simulink model "Model_Compare"  (R2018a)
settings: Solver=FixedStepDiscrete  StartTime=0.0  StopTime=37  FixedStep=Ts  RelTol=1e-3  EnableMultiTasking=on
values from neighbouring files (symbols this model uses):
  alpha_f0 = states(7)    [IS_2impulse.m]    (also in IS_3impulse.m; IS_4impulse.m; InputShaper.m; InputShaper2.m = 0)
  alpha_r0 = states(8)    [IS_2impulse.m]    (also in IS_3impulse.m; IS_4impulse.m; InputShaper.m; InputShaper2.m = 0)
  Bx_ash_f = 11.7    [ISData.m]    (also in SbWdata.m; pacjeka_params.m)
  Bx_ash_r = 11.1    [ISData.m]    (also in SbWdata.m; pacjeka_params.m)
  Bx_snow_f = 10.2    [ISData.m]    (also in SbWdata.m; pacjeka_params.m)
  Bx_snow_r = 9.71    [ISData.m]    (also in SbWdata.m; pacjeka_params.m)
  Bx_wash_f = 12    [ISData.m]    (also in SbWdata.m; pacjeka_params.m)
  Bx_wash_r = 11.5    [ISData.m]    (also in SbWdata.m; pacjeka_params.m)
  By_ash_f = 8.86    [ISData.m]    (also in SbWdata.m; pacjeka_params.m)
  By_ash_r = 9.30    (= 9.3)    [ISData.m]    (also in SbWdata.m; pacjeka_params.m)
  By_snow_f = 19.1    [ISData.m]    (also in SbWdata.m; pacjeka_params.m)
  By_snow_r = 20.0    (= 20)    [ISData.m]    (also in SbWdata.m; pacjeka_params.m)
  By_wash_f = 10.7    [ISData.m]    (also in SbWdata.m; pacjeka_params.m)
  By_wash_r = 11.3    [ISData.m]    (also in SbWdata.m; pacjeka_params.m)
  Cx_ash_f = 1.69    [ISData.m]    (also in SbWdata.m; pacjeka_params.m)
  Cx_ash_r = 1.69    [ISData.m]    (also in SbWdata.m; pacjeka_params.m)
  Cx_snow_f = 1.96    [ISData.m]    (also in SbWdata.m; pacjeka_params.m)
  Cx_snow_r = 1.96    [ISData.m]    (also in SbWdata.m; pacjeka_params.m)
  Cx_wash_f = 1.80    (= 1.8)    [ISData.m]    (also in SbWdata.m; pacjeka_params.m)
  Cx_wash_r = 1.80    (= 1.8)    [ISData.m]    (also in SbWdata.m; pacjeka_params.m)
  Cy_ash_f = 1.19    [ISData.m]    (also in SbWdata.m; pacjeka_params.m)
  Cy_ash_r = 1.19    [ISData.m]    (also in SbWdata.m; pacjeka_params.m)
  Cy_snow_f = 0.550    (= 0.55)    [ISData.m]    (also in SbWdata.m; pacjeka_params.m)
  Cy_snow_r = 0.550    (= 0.55)    [ISData.m]    (also in SbWdata.m; pacjeka_params.m)
  Cy_wash_f = 1.07    [ISData.m]    (also in SbWdata.m; pacjeka_params.m)
  Cy_wash_r = 1.07    [ISData.m]    (also in SbWdata.m; pacjeka_params.m)
  D_phi = 16000    [ISData.m]    (also in IS_2impulse.m; IS_3impulse.m; IS_4impulse.m; InputShaper.m)
  D_theta = 30960    [ISData.m]    (also in IS_2impulse.m; IS_3impulse.m; IS_4impulse.m; InputShaper.m)
  delta_r = 0    [ISData.m]    (also in IS_2impulse.m; IS_3impulse.m; IS_4impulse.m; InputShaper.m)
  epsilon = 0.4    [ISData.m]    (also in IS_2impulse.m; IS_3impulse.m; IS_4impulse.m; InputShaper.m)
  Ex_ash_f = 0.377    [ISData.m]    (also in SbWdata.m; pacjeka_params.m)
  Ex_ash_r = 0.362    [ISData.m]    (also in SbWdata.m; pacjeka_params.m)
  Ex_snow_f = 0.651    [ISData.m]    (also in SbWdata.m; pacjeka_params.m)
  Ex_snow_r = 0.624    [ISData.m]    (also in SbWdata.m; pacjeka_params.m)
  Ex_wash_f = 0.313    [ISData.m]    (also in SbWdata.m; pacjeka_params.m)
  Ex_wash_r = 0.300    (= 0.3)    [ISData.m]    (also in SbWdata.m; pacjeka_params.m)
  Ey_ash_f = -1.21    [ISData.m]    (also in SbWdata.m; pacjeka_params.m)
  Ey_ash_r = -1.11    [ISData.m]    (also in SbWdata.m; pacjeka_params.m)
  Ey_snow_f = -2.1    [ISData.m]    (also in SbWdata.m; pacjeka_params.m)
  Ey_snow_r = -1.93    [ISData.m]    (also in SbWdata.m; pacjeka_params.m)
  Ey_wash_f = -2.14    [ISData.m]    (also in SbWdata.m; pacjeka_params.m)
  Ey_wash_r = -1.97    [ISData.m]    (also in SbWdata.m; pacjeka_params.m)
  g = 9.81    [ISData.m]    (also in IS_2impulse.m; IS_3impulse.m; IS_4impulse.m; InputShaper.m)
  h = 0.5    [ISData.m]    (also in IS_2impulse.m; IS_3impulse.m; IS_4impulse.m; InputShaper.m)
  Iw = 4    [ISData.m]    (also in IS_2impulse.m; IS_3impulse.m; IS_4impulse.m; InputShaper.m)
  Ixx = 602.1923    [ISData.m]    (also in IS_2impulse.m; IS_3impulse.m; IS_4impulse.m; InputShaper.m)
  Iyy = 2.7370e+03    (= 2737)    [ISData.m]    (also in IS_2impulse.m; IS_3impulse.m; IS_4impulse.m; InputShaper.m)
  Iz = Izz    (= 3070)    [IS_2impulse.m]    (also in IS_3impulse.m; IS_4impulse.m; InputShaper.m; InputShaper2.m)
  Izz = 3070    [ISData.m]    (also in IS_2impulse.m; IS_3impulse.m; IS_4impulse.m; InputShaper.m)
  K_phi = 178000    [ISData.m]    (also in IS_2impulse.m; IS_3impulse.m; IS_4impulse.m; InputShaper.m)
  K_theta = 363540    [ISData.m]    (also in IS_2impulse.m; IS_3impulse.m; IS_4impulse.m; InputShaper.m)
  l = l_f+l_r    (= 2.67)    [IS_2impulse.m]    (also in IS_3impulse.m; IS_4impulse.m; InputShaper.m; InputShaper2.m)
  l_f = 1.2110    (= 1.211)    [ISData.m]    (also in IS_2impulse.m; IS_3impulse.m; IS_4impulse.m; InputShaper.m)
  l_r = 1.4590    (= 1.459)    [ISData.m]    (also in IS_2impulse.m; IS_3impulse.m; IS_4impulse.m; InputShaper.m)
  m = 1830    [ISData.m]    (also in IS_2impulse.m; IS_3impulse.m; IS_4impulse.m; InputShaper.m)
  mu_x_ash_f = 1.20    (= 1.2)    [ISData.m]    (also in SbWdata.m; pacjeka_params.m)
  mu_x_ash_r = 1.20    (= 1.2)    [ISData.m]    (also in SbWdata.m; pacjeka_params.m)
  mu_x_snow_f = 0.407    [ISData.m]    (also in SbWdata.m; pacjeka_params.m)
  mu_x_snow_r = 0.409    [ISData.m]    (also in SbWdata.m; pacjeka_params.m)
  mu_x_wash_f = 1.06    [ISData.m]    (also in SbWdata.m; pacjeka_params.m)
  mu_x_wash_r = 1.07    [ISData.m]    (also in SbWdata.m; pacjeka_params.m)
  mu_y_ash_f = 0.935    [ISData.m]    (also in SbWdata.m; pacjeka_params.m)
  mu_y_ash_r = 0.961    [ISData.m]    (also in SbWdata.m; pacjeka_params.m)
  mu_y_snow_f = 0.383    [ISData.m]    (also in SbWdata.m; pacjeka_params.m)
  mu_y_snow_r = 0.394    [ISData.m]    (also in SbWdata.m; pacjeka_params.m)
  mu_y_wash_f = 0.885    [ISData.m]    (also in SbWdata.m; pacjeka_params.m)
  mu_y_wash_r = 0.911    [ISData.m]    (also in SbWdata.m; pacjeka_params.m)
  omega0 = Vx0/Rw    (= 48.6005830904)    [ISData.m]    (also in IS_2impulse.m = 74.1; IS_3impulse.m = 74.1; IS_4impulse.m = 74.1; InputShaper.m = 55.5666666667)
  omega_f0 = states(5)    [IS_2impulse.m]    (also in IS_3impulse.m; IS_4impulse.m; InputShaper.m; InputShaper2.m = 55.5666666667)
  omega_r0 = states(6)    [IS_2impulse.m]    (also in IS_3impulse.m; IS_4impulse.m; InputShaper.m; InputShaper2.m = 55.5666666667)
  psi0 = states(2)    [IS_2impulse.m]    (also in IS_3impulse.m; IS_4impulse.m; InputShaper.m; InputShaper2.m = 0)
  psi_dot0 = states(1)    [IS_2impulse.m]    (also in IS_3impulse.m; IS_4impulse.m; InputShaper.m; InputShaper2.m = 0)
  Px0 = states(9)    [IS_2impulse.m]    (also in IS_3impulse.m; IS_4impulse.m; InputShaper.m; InputShaper2.m = 0)
  Py0 = states(10)    [IS_2impulse.m]    (also in IS_3impulse.m; IS_4impulse.m; InputShaper.m; InputShaper2.m = 0)
  Re = Rw    (= 0.3)    [IS_2impulse.m]    (also in IS_3impulse.m; IS_4impulse.m; InputShaper.m; InputShaper2.m)
  road = 1    [ISData.m]    (also in IS_2impulse.m; IS_3impulse.m; IS_4impulse.m; InputShaper.m)
  Rw = 0.3430    (= 0.343)    [ISData.m]    (also in IS_2impulse.m = 0.3; IS_3impulse.m = 0.3; IS_4impulse.m = 0.3; InputShaper.m = 0.3)
  sigma = epsilon    (= 0.4)    [IS_2impulse.m]    (also in IS_3impulse.m; IS_4impulse.m; InputShaper.m; InputShaper2.m)
  Ts = 0.001    [ISData.m]    (also in IS_2impulse.m; IS_3impulse.m; IS_4impulse.m; InputShaper.m)
  Tsmall = 0.001    [ISData.m]    (also in IS_2impulse.m; IS_3impulse.m; IS_4impulse.m; InputShaper.m)
  Vx0 = 16.67    [ISData.m]    (also in IS_2impulse.m = states(3); IS_3impulse.m = states(3); IS_4impulse.m = states(3); InputShaper.m = states(3))
  Vy0 = states(4)    [IS_2impulse.m]    (also in IS_3impulse.m; IS_4impulse.m; InputShaper.m; InputShaper2.m = 0)
  w = 0.7700    (= 0.77)    [ISData.m]    (also in IS_2impulse.m; IS_3impulse.m; IS_4impulse.m; InputShaper.m)
undefined symbols (not defined in the file or in its folder): theta_sw_FH
libraries: simulink x2
(part 3 of 3)

== system Model_Compare/3DoF_Vehicle1/Subsystem1/Pacjeka_parameters_Subsystem/WetAshphalt_condition_subsystem ==
  Action Port : ActionPort  ActionType=case
  Bx_wash_f : Constant  Value=Bx_wash_f
  Bx_wash_r : Constant  Value=Bx_wash_r
  By_wash_f : Constant  Value=By_wash_f
  By_wash_r : Constant  Value=By_wash_r
  Cx_wash_f : Constant  Value=Cx_wash_f
  Cx_wash_r : Constant  Value=Cx_wash_r
  Cy_wash_f : Constant  Value=Cy_wash_f
  Cy_wash_r : Constant  Value=Cy_wash_r
  Ex_wash_f : Constant  Value=Ex_wash_f
  Ex_wash_r : Constant  Value=Ex_wash_r
  Ey_wash_f : Constant  Value=Ey_wash_f
  Ey_wash_r : Constant  Value=Ey_wash_r
  Mux : Mux  Inputs=16
      settings: DisplayOption=signals
  mu_x_wash_f : Constant  Value=mu_x_wash_f
  mu_x_wash_r : Constant  Value=mu_x_wash_r
  mu_y_wash_f : Constant  Value=mu_y_wash_f
  mu_y_wash_r : Constant  Value=mu_y_wash_r
  Out1 : Outport  OutDataTypeStr=double  SampleTime=Ts
  wires:
  mu_x_wash_f/1 -> Mux/1  "mu_x_wash_f"
  mu_y_wash_f/1 -> Mux/2  "mu_y_wash_f"
  Cx_wash_f/1 -> Mux/3  "Cx_wash_f"
  Cy_wash_f/1 -> Mux/4  "Cy_wash_f"
  Bx_wash_f/1 -> Mux/5  "Bx_wash_f"
  By_wash_f/1 -> Mux/6  "By_wash_f"
  Ex_wash_f/1 -> Mux/7  "Ex_wash_f"
  Ey_wash_f/1 -> Mux/8  "E_y_wash_f"
  Cy_wash_r/1 -> Mux/12  "Cy_wash_r"
  Cx_wash_r/1 -> Mux/11  "Cx_wash_r"
  By_wash_r/1 -> Mux/14  "By_wash_r"
  Bx_wash_r/1 -> Mux/13  "Bx_wash_r"
  mu_y_wash_r/1 -> Mux/10  "mu_y_wash_r"
  Ex_wash_r/1 -> Mux/15  "Ex_wash_r"
  mu_x_wash_r/1 -> Mux/9  "mu_x_wash_r"
  Ey_wash_r/1 -> Mux/16  "Ey_wash_r"
  Mux/1 -> Out1/1

== system Model_Compare/3DoF_Vehicle1/Subsystem1/Vxdot_subsystem/Fy_subsystem ==
  Fyf : Inport
  Fxf : Inport  Port=2
  Fxr : Inport  Port=3
  cosDelta : Inport  Port=4
  sinDelta : Inport  Port=5
  Add : Sum
  Mux : Mux  Inputs=3
  Terminator : Terminator
  Fx : Outport
  wires:
  Add/1 -> Fx/1
  Fxf/1 -> Add/1
  Fxr/1 -> Add/2
  Mux/1 -> Terminator/1
  cosDelta/1 -> Mux/1
  sinDelta/1 -> Mux/2
  Fyf/1 -> Mux/3

== system Model_Compare/3DoF_Vehicle1/Subsystem1/Vydot_subsystem/Fy_subsystem ==
  Fyf : Inport
  Fyr : Inport  Port=2
  Fxf : Inport  Port=3
  cosDelta : Inport  Port=4
  sinDelta : Inport  Port=5
  Add : Sum  Inputs=2
  Mux : Mux  Inputs=3
  Terminator : Terminator
  Fy : Outport
  wires:
  Add/1 -> Fy/1
  Fyf/1 -> Add/1
  Fyr/1 -> Add/2
  Fxf/1 -> Mux/1
  cosDelta/1 -> Mux/2
  sinDelta/1 -> Mux/3
  Mux/1 -> Terminator/1

== system Model_Compare/Vehicle_Sim/Vehicle_model/Fz_Subsystem/tau_phi_subsystem ==
  K_phi : Inport
  D_phi : Inport  Port=2
  phi_dot : Inport  Port=3
  phi : Inport  Port=4
  Add : Sum
  Add1 : Sum
  Divide{,1..3} (4 alike) : Product  Inputs=**
  Gain : Gain  Gain=0.5
  Gain1 : Gain  Gain=0.5
  tau_phi_f : Outport
  tau_phi_r : Outport  Port=2
  wires:
  Divide2/1 -> Add1/1
  Divide/1 -> Add/1
  Add/1 -> tau_phi_f/1  "tau_phi_f"
  Divide1/1 -> Add/2
  Gain1/1 -> Divide3/1, Divide1/1  "D_phi_r"
  Gain/1 -> Divide2/1, Divide/1  "K_phi_r"
  D_phi/1 -> Gain1/1
  phi/1 -> Divide2/2, Divide/2  "phi"
  Divide3/1 -> Add1/2
  phi_dot/1 -> Divide3/2, Divide1/2  "phi_dot"
  K_phi/1 -> Gain/1
  Add1/1 -> tau_phi_r/1  "tau_phi_r"

== system Model_Compare/Vehicle_Sim/Vehicle_model/Fz_Subsystem/tau_theta_subsystem ==
  theta_dot : Inport  OutDataTypeStr=double  SampleTime=Ts  LockScale=on
  theta : Inport  Port=2  OutDataTypeStr=double  SampleTime=Ts
  K_theta : Inport  Port=3  OutDataTypeStr=double  SampleTime=Ts
  D_theta : Inport  Port=4  OutDataTypeStr=double  SampleTime=Ts
  Add : Sum
  Divide : Product  Inputs=**
  Divide1 : Product  Inputs=**
  tau_theta : Outport  OutDataTypeStr=double  SampleTime=Ts
  wires:
  Add/1 -> tau_theta/1
  Divide/1 -> Add/1
  Divide1/1 -> Add/2
  K_theta/1 -> Divide/1
  D_theta/1 -> Divide1/2
  theta_dot/1 -> Divide1/1
  theta/1 -> Divide/2

== system Model_Compare/Vehicle_Sim/Vehicle_model/Pacjeka_parameters_Subsystem/Ashphalt_condition_subsystem ==
  Action Port : ActionPort  ActionType=then
  Bx_ash_f : Constant  Value=Bx_ash_f
  Bx_ash_r : Constant  Value=Bx_ash_r
  By_ash_f : Constant  Value=By_ash_f
  By_ash_r : Constant  Value=By_ash_r
  Cx_ash_f : Constant  Value=Cx_ash_f
  Cx_ash_r : Constant  Value=Cx_ash_r
  Cy_ash_f : Constant  Value=Cy_ash_f
  Cy_ash_r : Constant  Value=Cy_ash_r
  Ex_ash_f : Constant  Value=Ex_ash_f
  Ex_ash_r : Constant  Value=Ex_ash_r
  Ey_ash_f : Constant  Value=Ey_ash_f
  Ey_ash_r : Constant  Value=Ey_ash_r
  Mux : Mux  Inputs=16
      settings: DisplayOption=signals
  mu_x_ash_f : Constant  Value=mu_x_ash_f
  mu_x_ash_r : Constant  Value=mu_x_ash_r
  mu_y_ash_f : Constant  Value=mu_y_ash_f
  mu_y_ash_r : Constant  Value=mu_y_ash_r
  Out1 : Outport  OutDataTypeStr=double  SampleTime=Ts
  wires:
  mu_x_ash_f/1 -> Mux/1  "mu_x_ash_f"
  mu_y_ash_f/1 -> Mux/2  "mu_y_ash_f"
  Cx_ash_f/1 -> Mux/3  "Cx_ash_f"
  Cy_ash_f/1 -> Mux/4  "Cy_ash_f"
  Bx_ash_f/1 -> Mux/5  "Bx_ash_f"
  By_ash_f/1 -> Mux/6  "By_ash_f"
  Ex_ash_f/1 -> Mux/7  "Ex_ash_f"
  Ey_ash_f/1 -> Mux/8  "E_y_ash_f"
  Cy_ash_r/1 -> Mux/12  "Cy_ash_r"
  Cx_ash_r/1 -> Mux/11  "Cx_ash_r"
  By_ash_r/1 -> Mux/14  "By_ash_r"
  Bx_ash_r/1 -> Mux/13  "Bx_ash_r"
  mu_y_ash_r/1 -> Mux/10  "mu_y_ash_r"
  Ex_ash_r/1 -> Mux/15  "Ex_ash_r"
  mu_x_ash_r/1 -> Mux/9  "mu_x_ash_r"
  Ey_ash_r/1 -> Mux/16  "Ey_ash_r"
  Mux/1 -> Out1/1

== system Model_Compare/Vehicle_Sim/Vehicle_model/Pacjeka_parameters_Subsystem/Snow_condition_subsystem ==
  Action Port : ActionPort  ActionType=else
  Bx_snow_f : Constant  Value=Bx_snow_f
  Bx_snow_r : Constant  Value=Bx_snow_r
  By_snow_f : Constant  Value=By_snow_f
  By_snow_r : Constant  Value=By_snow_r
  Cx_snow_f : Constant  Value=Cx_snow_f
  Cx_snow_r : Constant  Value=Cx_snow_r
  Cy_snow_f : Constant  Value=Cy_snow_f
  Cy_snow_r : Constant  Value=Cy_snow_r
  Ex_snow_f : Constant  Value=Ex_snow_f
  Ex_snow_r : Constant  Value=Ex_snow_r
  Ey_snow_f : Constant  Value=Ey_snow_f
  Ey_snow_r : Constant  Value=Ey_snow_r
  Mux : Mux  Inputs=16
  mu_x_snow_f : Constant  Value=mu_x_snow_f
  mu_x_snow_r : Constant  Value=mu_x_snow_r
  mu_y_snow_f : Constant  Value=mu_y_snow_f
  mu_y_snow_r : Constant  Value=mu_y_snow_r
  Out1 : Outport  OutDataTypeStr=double  SampleTime=Ts
  wires:
  Ex_snow_r/1 -> Mux/15
  Cy_snow_r/1 -> Mux/12
  By_snow_r/1 -> Mux/14
  Cx_snow_r/1 -> Mux/11
  mu_y_snow_r/1 -> Mux/10
  mu_x_snow_r/1 -> Mux/9
  Bx_snow_r/1 -> Mux/13
  Ey_snow_r/1 -> Mux/16
  mu_x_snow_f/1 -> Mux/1
  mu_y_snow_f/1 -> Mux/2
  Cx_snow_f/1 -> Mux/3
  Cy_snow_f/1 -> Mux/4
  Bx_snow_f/1 -> Mux/5
  By_snow_f/1 -> Mux/6
  Ex_snow_f/1 -> Mux/7
  Ey_snow_f/1 -> Mux/8
  Mux/1 -> Out1/1

== system Model_Compare/Vehicle_Sim/Vehicle_model/omega_alpha_and_k_values_subsystem/Subsystem ==
  Vx1 : Inport  OutDataTypeStr=double  SampleTime=Ts
  Vy1 : Inport  Port=2  OutDataTypeStr=double  SampleTime=Ts
  epsilon : Inport  Port=3  OutDataTypeStr=double  SampleTime=Ts
  apha_f1_curr : Inport  Port=4  OutDataTypeStr=double  SampleTime=Tsmall
  Add : Sum  Inputs=+-
  Add1 : Sum
  Divide : Product  Inputs=*/
  Divide1 : Product  Inputs=*/
  Gain : Gain  Gain=-1
  Gain1 : Gain  Gain=Tsmall
  Product : Product
  Product1 : Product
  Trigonometric Function : Trigonometry  Operator=atan
  alpha_f1_next : Outport  OutDataTypeStr=double  SampleTime=Tsmall
  wires:
  Gain1/1 -> Add1/1  "alpha_f1dot*Tsmall"
  Vx1/1 -> Divide1/2, Divide/1
  Product1/1 -> Add/2
  Divide1/1 -> Trigonometric Function/1
  Divide/1 -> Gain/1, Product1/1
  Product/1 -> Add/1
  epsilon/1 -> Divide/2
  Trigonometric Function/1 -> Product/2
  Vy1/1 -> Divide1/1
  Add/1 -> Gain1/1  "alpha_f1_dot"
  Gain/1 -> Product/1
  Add1/1 -> alpha_f1_next/1
  apha_f1_curr/1 -> Add1/2, Product1/2

== system Model_Compare/Vehicle_Sim/Vehicle_model/omega_alpha_and_k_values_subsystem/Subsystem1 ==
  Vx2 : Inport  OutDataTypeStr=double  SampleTime=Ts
  Vy2 : Inport  Port=2  OutDataTypeStr=double  SampleTime=Ts
  epsilon : Inport  Port=3  OutDataTypeStr=double  SampleTime=Ts
  alpha_f2_curr : Inport  Port=4  OutDataTypeStr=double  SampleTime=Tsmall
  Add : Sum  Inputs=+-
  Add1 : Sum
  Divide : Product  Inputs=*/
  Divide1 : Product  Inputs=*/
  Gain : Gain  Gain=-1
  Gain1 : Gain  Gain=Tsmall
  Product : Product
  Product1 : Product
  Trigonometric Function : Trigonometry  Operator=atan
  alpha_f2_next : Outport  OutDataTypeStr=double  SampleTime=Tsmall
  wires:
  Gain1/1 -> Add1/1  "alpha_f2dot*Tsmall"
  Vx2/1 -> Divide1/2, Divide/1
  Product1/1 -> Add/2
  Divide1/1 -> Trigonometric Function/1
  Divide/1 -> Gain/1, Product1/1
  Product/1 -> Add/1
  epsilon/1 -> Divide/2
  Trigonometric Function/1 -> Product/2
  Vy2/1 -> Divide1/1
  Add/1 -> Gain1/1  "alpha_f2_dot"
  Gain/1 -> Product/1
  alpha_f2_curr/1 -> Add1/2, Product1/2
  Add1/1 -> alpha_f2_next/1

== system Model_Compare/Vehicle_Sim/Vehicle_model/omega_alpha_and_k_values_subsystem/Subsystem2 ==
  Vx3 : Inport  OutDataTypeStr=double  SampleTime=Ts
  Vy3 : Inport  Port=2  OutDataTypeStr=double  SampleTime=Ts
  epsilon : Inport  Port=3  OutDataTypeStr=double  SampleTime=Ts
  alpha_r3_curr : Inport  Port=4  OutDataTypeStr=double  SampleTime=Tsmall
  Add : Sum  Inputs=+-
  Add1 : Sum
  Divide : Product  Inputs=*/
  Divide1 : Product  Inputs=*/
  Gain : Gain  Gain=-1
  Gain1 : Gain  Gain=Tsmall
  Product : Product
  Product1 : Product
  Trigonometric Function : Trigonometry  Operator=atan
  alpha_r3_next : Outport  OutDataTypeStr=double  SampleTime=Tsmall
  wires:
  Gain1/1 -> Add1/1  "alpha_r3dot*Tsmall"
  Vx3/1 -> Divide1/2, Divide/1
  Product1/1 -> Add/2
  Divide1/1 -> Trigonometric Function/1
  Divide/1 -> Gain/1, Product1/1
  Product/1 -> Add/1
  epsilon/1 -> Divide/2
  Trigonometric Function/1 -> Product/2
  Vy3/1 -> Divide1/1
  Add/1 -> Gain1/1  "alpha_r3_dot"
  Gain/1 -> Product/1
  alpha_r3_curr/1 -> Add1/2, Product1/2
  Add1/1 -> alpha_r3_next/1

== system Model_Compare/Vehicle_Sim/Vehicle_model/omega_alpha_and_k_values_subsystem/Subsystem3 ==
  Vx4 : Inport  OutDataTypeStr=double  SampleTime=Ts
  Vy4 : Inport  Port=2  OutDataTypeStr=double  SampleTime=Ts
  epsilon : Inport  Port=3  OutDataTypeStr=double  SampleTime=Ts
  alpha_r4_curr : Inport  Port=4  OutDataTypeStr=double  SampleTime=Tsmall
  Add : Sum  Inputs=+-
  Add1 : Sum
  Divide : Product  Inputs=*/
  Divide1 : Product  Inputs=*/
  Gain : Gain  Gain=-1
  Gain1 : Gain  Gain=Tsmall
  Product : Product
  Product1 : Product
  Trigonometric Function : Trigonometry  Operator=atan
  alpha_r4_next : Outport  OutDataTypeStr=double  SampleTime=Tsmall
  wires:
  Gain1/1 -> Add1/1  "alpha_r4dot*Tsmall"
  Vx4/1 -> Divide1/2, Divide/1
  Product1/1 -> Add/2
  Divide1/1 -> Trigonometric Function/1
  Divide/1 -> Gain/1, Product1/1
  Product/1 -> Add/1
  epsilon/1 -> Divide/2
  Trigonometric Function/1 -> Product/2
  Vy4/1 -> Divide1/1
  Add/1 -> Gain1/1  "alpha_r4_dot"
  Gain/1 -> Product/1
  alpha_r4_curr/1 -> Add1/2, Product1/2
  Add1/1 -> alpha_r4_next/1

== system Model_Compare/Vehicle_Sim/Vehicle_model/omega_alpha_and_k_values_subsystem/Subsystem4 ==
  T1 : Inport  OutDataTypeStr=double  SampleTime=Ts
  T2 : Inport  Port=2  OutDataTypeStr=double  SampleTime=Ts
  T3 : Inport  Port=3  OutDataTypeStr=double  SampleTime=Ts
  T4 : Inport  Port=4  OutDataTypeStr=double  SampleTime=Ts
  Iw : Inport  Port=5  OutDataTypeStr=double  SampleTime=Ts
  Fx1 : Inport  Port=6  OutDataTypeStr=double  SampleTime=Ts
  Fx2 : Inport  Port=7  OutDataTypeStr=double  SampleTime=Ts
  Fx3 : Inport  Port=8  OutDataTypeStr=double  SampleTime=Ts
  Fx4 : Inport  Port=9  OutDataTypeStr=double  SampleTime=Ts
  Rw : Inport  Port=10  OutDataTypeStr=double  SampleTime=Ts
  Add{4..7} (4 alike) : Sum  Inputs=+-
  Divide{4..7} (4 alike) : Product  Inputs=*/
  Product{4..7} (4 alike) : Product
  omega_dot1 : Outport  OutDataTypeStr=double  SampleTime=Tsmall
  omega_dot2 : Outport  Port=2  OutDataTypeStr=double  SampleTime=Tsmall
  omega_dot3 : Outport  Port=3  OutDataTypeStr=double  SampleTime=Tsmall
  omega_dot4 : Outport  Port=4  OutDataTypeStr=double  SampleTime=Tsmall
  wires:
  Product7/1 -> Add7/2
  Add7/1 -> Divide7/1
  Iw/1 -> Divide7/2, Divide6/2, Divide5/2, Divide4/2
  Add5/1 -> Divide5/1
  T1/1 -> Add4/1
  Product5/1 -> Add5/2
  Rw/1 -> Product4/2, Product5/2, Product7/2, Product6/2
  Divide7/1 -> omega_dot4/1  "omega_dot4"
  Fx3/1 -> Product6/1
  Add4/1 -> Divide4/1
  Fx2/1 -> Product5/1
  T4/1 -> Add7/1
  Fx1/1 -> Product4/1
  T3/1 -> Add6/1
  Product4/1 -> Add4/2
  T2/1 -> Add5/1
  Product6/1 -> Add6/2
  Add6/1 -> Divide6/1
  Fx4/1 -> Product7/1
  Divide6/1 -> omega_dot3/1  "omega_dot3"
  Divide5/1 -> omega_dot2/1  "omega_dot2"
  Divide4/1 -> omega_dot1/1  "omega_dot1"

== system Model_Compare/Vehicle_Sim/Vehicle_model/omega_alpha_and_k_values_subsystem/Subsystem5 ==
  Vx : Inport  OutDataTypeStr=double  SampleTime=Ts
  w : Inport  Port=2  OutDataTypeStr=double  SampleTime=Ts
  delta_f2 : Inport  Port=3  OutDataTypeStr=double  SampleTime=Ts
  Vy : Inport  Port=4  OutDataTypeStr=double  SampleTime=Ts
  l_f : Inport  Port=5  OutDataTypeStr=double  SampleTime=Ts
  l_r : Inport  Port=6  OutDataTypeStr=double  SampleTime=Ts
  psi_dot : Inport  Port=7  OutDataTypeStr=double  SampleTime=Ts
  Add : Sum
  Add1 : Sum
  Add2 : Sum  Inputs=-+
  Constant : Constant  Value=delta_r
  Cos : Trigonometry  Operator=cos
  Cos1 : Trigonometry  Operator=cos
  Gain{,1..3} (4 alike) : Gain
  Multiply : Product
  Multiply1 : Product
  Multiply2 : Product
  Subsystem : Subsystem
  Subsystem1 : Subsystem
  Subsystem2 : Subsystem
  Subsystem3 : Subsystem
  Subtract : Sum  Inputs=+-
  sin : Trigonometry
  sin1 : Trigonometry
  Vx1 : Outport  OutDataTypeStr=double  SampleTime=Ts
  Vx2 : Outport  Port=2  OutDataTypeStr=double  SampleTime=Ts
  Vx3 : Outport  Port=3  OutDataTypeStr=double  SampleTime=Ts
  Vx4 : Outport  Port=4  OutDataTypeStr=double  SampleTime=Ts
  Vy1 : Outport  Port=5  OutDataTypeStr=double  SampleTime=Ts
  Vy2 : Outport  Port=6  OutDataTypeStr=double  SampleTime=Ts
  Vy3 : Outport  Port=7  OutDataTypeStr=double  SampleTime=Ts
  Vy4 : Outport  Port=8  OutDataTypeStr=double  SampleTime=Ts
  wires:
  delta_f2/1 -> Cos/1, sin/1
  Constant/1 -> sin1/1, Cos1/1
  Vy/1 -> Add2/2, Add1/2  "Vy"
  Vx/1 -> Add/1, Subtract/1  "Vx"
  psi_dot/1 -> Multiply1/2, Multiply2/1, Multiply/1  "psi_dot"
  l_f/1 -> Multiply/2
  Multiply/1 -> Add1/1  "l_f*psi_dot"
  w/1 -> Multiply1/1
  Multiply1/1 -> Add/2, Subtract/2  "w*psi_dot"
  l_r/1 -> Multiply2/2
  Multiply2/1 -> Add2/1  "l_r*psi_dot"
  Subtract/1 -> Subsystem/1(Vx1_ur), Gain/1  "Vx1_ur"
  Add/1 -> Subsystem1/1(Vx2_ur), Gain1/1  "Vx2_ur"
  Add1/1 -> Gain2/1, Subsystem/2(Vy1_ur)  "Vy1_ur"
  Add2/1 -> Subsystem2/4(Vy3_ur), Gain3/1  "Vy3_ur"
  Cos/1 -> Subsystem1/3(cosDeltaf2), Subsystem/3(cosDeltaf2)  "cosDeltaf2"
  sin/1 -> Subsystem1/4(sinDeltaf2), Subsystem/4(sinDeltaf2)  "sinDeltaf2"
  Gain2/1 -> Subsystem1/2(Vy2_ur)  "Vy2_ur"
  Cos1/1 -> Subsystem3/1(cosDelta_r), Subsystem2/1(cosDelta_r)  "cosDelta_r"
  sin1/1 -> Subsystem3/2(sinDelta_r), Subsystem2/2(sinDelta_r)  "sinDelta_r"
  Gain/1 -> Subsystem2/3(Vx3_ur)  "Vx3_ur"
  Gain1/1 -> Subsystem3/3(Vx4_ur)  "Vx4_ur"
  Gain3/1 -> Subsystem3/4(Vy4_ur)  "Vy4_ur"
  Subsystem2/1(Vx3) -> Vx3/1
  Subsystem2/2(Vy3) -> Vy3/1
  Subsystem3/1(Vx4) -> Vx4/1
  Subsystem3/2(Vy4) -> Vy4/1
  Subsystem/1(Vx1) -> Vx1/1
  Subsystem/2(Vy1) -> Vy1/1
  Subsystem1/1(Vx2) -> Vx2/1
  Subsystem1/2(Vy2) -> Vy2/1

== system Model_Compare/Vehicle_Sim/Vehicle_model/phi_subsystem/phi_ddot_denominator_subsystem ==
  phi : Inport  OutDataTypeStr=double  SampleTime=Tsmall
  theta : Inport  Port=2  OutDataTypeStr=double  SampleTime=Tsmall
  Ixx : Inport  Port=3  OutDataTypeStr=double  SampleTime=Ts
  Iyy : Inport  Port=4  OutDataTypeStr=double  SampleTime=Ts
  Izz : Inport  Port=5  OutDataTypeStr=double  SampleTime=Ts
  Add : Sum  Inputs=+++
  Divide : Product  Inputs=**
  Divide1 : Product  Inputs=***
  Divide2 : Product  Inputs=***
  Square{,1..3} (4 alike) : Math  Operator=square  RndMeth=Zero  SaturateOnIntegerOverflow=on
  Trigonometric Function : Trigonometry  Operator=cos
  Trigonometric Function1 : Trigonometry
  Trigonometric Function2 : Trigonometry
  Trigonometric Function3 : Trigonometry  Operator=cos
  phi_ddot_denominator : Outport  OutDataTypeStr=double  SampleTime=Tsmall
  wires:
  Trigonometric Function1/1 -> Square1/1
  Iyy/1 -> Divide1/2
  Square1/1 -> Divide2/1, Divide1/1
  Square3/1 -> Divide2/2
  Square2/1 -> Divide1/3
  phi/1 -> Trigonometric Function2/1, Trigonometric Function3/1
  theta/1 -> Trigonometric Function1/1, Trigonometric Function/1
  Divide2/1 -> Add/3
  Divide/1 -> Add/1
  Add/1 -> phi_ddot_denominator/1
  Trigonometric Function3/1 -> Square3/1
  Izz/1 -> Divide2/3
  Square/1 -> Divide/1
  Trigonometric Function/1 -> Square/1
  Divide1/1 -> Add/2
  Ixx/1 -> Divide/2
  Trigonometric Function2/1 -> Square2/1

== system Model_Compare/Vehicle_Sim/Vehicle_model/phi_subsystem/phi_ddot_numerator_subsystem ==
  FY : Inport  OutDataTypeStr=double  SampleTime=Ts
  psi_dot : Inport  Port=2  OutDataTypeStr=double  SampleTime=Tsmall
  phi_dot : Inport  Port=3  OutDataTypeStr=double  SampleTime=Tsmall
  phi : Inport  Port=4  OutDataTypeStr=double  SampleTime=Tsmall
  theta_dot : Inport  Port=5  OutDataTypeStr=double  SampleTime=Tsmall
  theta : Inport  Port=6  OutDataTypeStr=double  SampleTime=Tsmall
  Iyy : Inport  Port=7  OutDataTypeStr=double  SampleTime=Ts
  Izz : Inport  Port=8  OutDataTypeStr=double  SampleTime=Ts
  K_phi : Inport  Port=9  OutDataTypeStr=double  SampleTime=Ts
  D_phi : Inport  Port=10  OutDataTypeStr=double  SampleTime=Ts
  h : Inport  Port=11  OutDataTypeStr=double  SampleTime=Ts
  Add : Sum
  Add1 : Sum  Inputs=+++
  Add2 : Sum
  Add3 : Sum  Inputs=+-
  Add4 : Sum
  Add7 : Sum  Inputs=+++
  Divide{,1..4,7..12} (11 alike) : Product  Inputs=**
  Divide5 : Product  Inputs=****
  Divide6 : Product  Inputs=****
  Gain : Gain  Gain=m*g
  Gain2 : Gain  Gain=-1
  Gain3 : Gain  Gain=-1
  Square : Math  Operator=square  RndMeth=Zero  SaturateOnIntegerOverflow=on
  Square1 : Math  Operator=square  RndMeth=Zero  SaturateOnIntegerOverflow=on
  Trigonometric Function : Trigonometry
  Trigonometric Function1 : Trigonometry  Operator=cos
  Trigonometric Function2 : Trigonometry  Operator=cos
  Trigonometric Function3 : Trigonometry
  phi_ddot_numerator : Outport  OutDataTypeStr=double  SampleTime=Tsmall
  wires:
  phi_dot/1 -> Divide1/1, Divide6/3  "phi_dot"
  psi_dot/1 -> Divide4/1, Divide5/4, Divide11/2  "psi_dot"
  Divide6/1 -> Add4/2
  phi/1 -> Divide/1, Trigonometric Function/1, Trigonometric Function1/1  "phi"
  theta/1 -> Trigonometric Function2/1, Trigonometric Function3/1  "theta"
  FY/1 -> Divide2/1  "FY"
  theta_dot/1 -> Divide11/1  "theta_dot"
  Gain2/1 -> Divide/2
  Gain3/1 -> Divide1/2
  Divide1/1 -> Add1/2
  Divide9/1 -> Add2/2
  Divide12/1 -> Add1/3
  Add/1 -> Divide12/1
  Divide3/1 -> Add/2
  Add2/1 -> Divide10/1
  Iyy/1 -> Divide9/2, Add3/1  "Iyy"
  Divide2/1 -> Divide3/1
  Square1/1 -> Divide8/2
  Izz/1 -> Add3/2, Divide8/1  "Izz"
  Add3/1 -> Divide4/2  "del_Iyz"
  Gain/1 -> Add/1
  Add7/1 -> phi_ddot_numerator/1
  Divide8/1 -> Add2/1
  Divide4/1 -> Divide7/1
  Add4/1 -> Divide7/2
  Trigonometric Function2/1 -> Divide3/2, Divide5/3  "cosTheta"
  Divide11/1 -> Divide10/2
  Divide5/1 -> Add4/1
  Divide7/1 -> Add7/2
  Square/1 -> Divide9/1
  Trigonometric Function1/1 -> Divide2/2, Divide5/2, Square/1, Divide6/2  "cosPhi"
  Divide10/1 -> Add7/3
  Add1/1 -> Add7/1
  Trigonometric Function3/1 -> Divide6/4  "sinTheta"
  Divide/1 -> Add1/1
  Trigonometric Function/1 -> Divide5/1, Divide6/1, Square1/1, Gain/1  "sinPhi"
  K_phi/1 -> Gain2/1  "K_phi"
  D_phi/1 -> Gain3/1  "D_phi"
  h/1 -> Divide12/2  "h"

== system Model_Compare/Vehicle_Sim/Vehicle_model/omega_alpha_and_k_values_subsystem/Subsystem5/Subsystem ==
  Vx1_ur : Inport
  Vy1_ur : Inport  Port=2
  cosDeltaf2 : Inport  Port=3
  sinDeltaf2 : Inport  Port=4
  Add3 : Sum
  Multiply{3..6} (4 alike) : Product
  Subtract1 : Sum  Inputs=+-
  Vx1 : Outport
  Vy1 : Outport  Port=2
  wires:
  Subtract1/1 -> Vy1/1  "Vy1"
  Multiply6/1 -> Add3/2
  Multiply5/1 -> Add3/1
  sinDeltaf2/1 -> Multiply4/2, Multiply6/2
  cosDeltaf2/1 -> Multiply3/2, Multiply5/2
  Vx1_ur/1 -> Multiply4/1, Multiply5/1
  Multiply3/1 -> Subtract1/1
  Vy1_ur/1 -> Multiply3/1, Multiply6/1
  Multiply4/1 -> Subtract1/2
  Add3/1 -> Vx1/1  "Vx1"

== system Model_Compare/Vehicle_Sim/Vehicle_model/omega_alpha_and_k_values_subsystem/Subsystem5/Subsystem1 ==
  Vx2_ur : Inport
  Vy2_ur : Inport  Port=2
  cosDeltaf2 : Inport  Port=3
  sinDeltaf2 : Inport  Port=4
  Add4 : Sum
  Multiply{7..10} (4 alike) : Product
  Subtract2 : Sum  Inputs=+-
  Vx2 : Outport
  Vy2 : Outport  Port=2
  wires:
  Vx2_ur/1 -> Multiply9/2, Multiply8/2
  sinDeltaf2/1 -> Multiply8/1, Multiply10/1
  Vy2_ur/1 -> Multiply10/2, Multiply7/2
  Add4/1 -> Vx2/1  "Vx2"
  Multiply10/1 -> Add4/2
  cosDeltaf2/1 -> Multiply7/1, Multiply9/1
  Multiply9/1 -> Add4/1
  Multiply8/1 -> Subtract2/2
  Multiply7/1 -> Subtract2/1
  Subtract2/1 -> Vy2/1  "Vy2"

== system Model_Compare/Vehicle_Sim/Vehicle_model/omega_alpha_and_k_values_subsystem/Subsystem5/Subsystem2 ==
  cosDelta_r : Inport
  sinDelta_r : Inport  Port=2
  Vx3_ur : Inport  Port=3
  Vy3_ur : Inport  Port=4
  Add3 : Sum
  Multiply{3..6} (4 alike) : Product
  Subtract1 : Sum  Inputs=+-
  Vx3 : Outport
  Vy3 : Outport  Port=2
  wires:
  Vy3_ur/1 -> Multiply3/1, Multiply6/2
  sinDelta_r/1 -> Multiply4/1, Multiply6/1
  Multiply3/1 -> Subtract1/1
  Multiply6/1 -> Add3/2
  Multiply4/1 -> Subtract1/2
  Multiply5/1 -> Add3/1
  Vx3_ur/1 -> Multiply4/2, Multiply5/2
  Add3/1 -> Vx3/1  "Vx3"
  cosDelta_r/1 -> Multiply3/2, Multiply5/1
  Subtract1/1 -> Vy3/1  "Vy3"

== system Model_Compare/Vehicle_Sim/Vehicle_model/omega_alpha_and_k_values_subsystem/Subsystem5/Subsystem3 ==
  cosDelta_r : Inport
  sinDelta_r : Inport  Port=2
  Vx4_ur : Inport  Port=3
  Vy4_ur : Inport  Port=4
  Add3 : Sum
  Multiply{3..6} (4 alike) : Product
  Subtract1 : Sum  Inputs=+-
  Vx4 : Outport
  Vy4 : Outport  Port=2
  wires:
  Multiply6/1 -> Add3/2
  Multiply5/1 -> Add3/1
  sinDelta_r/1 -> Multiply4/1, Multiply6/1
  Vy4_ur/1 -> Multiply6/2, Multiply3/2
  Add3/1 -> Vx4/1  "Vx4"
  Multiply4/1 -> Subtract1/2
  Multiply3/1 -> Subtract1/1
  Subtract1/1 -> Vy4/1  "Vy4"
  cosDelta_r/1 -> Multiply5/1, Multiply3/1
  Vx4_ur/1 -> Multiply4/2, Multiply5/2

== matlab function Model_Compare/MATLAB Function ==
  data: theta_sw_FH input; y output; T input
function y = fcn(theta_sw_FH,T)
    i=(T+0.001)/0.001;
    
y = theta_sw_FH(i);
